simulink model "propellantmassfunction"  (R2025b)
settings: Solver=VariableStepAuto  StartTime=0.0  StopTime=10.0  RelTol=1e-3
settings Model: Creator=zachm  LastModifiedBy=zachm

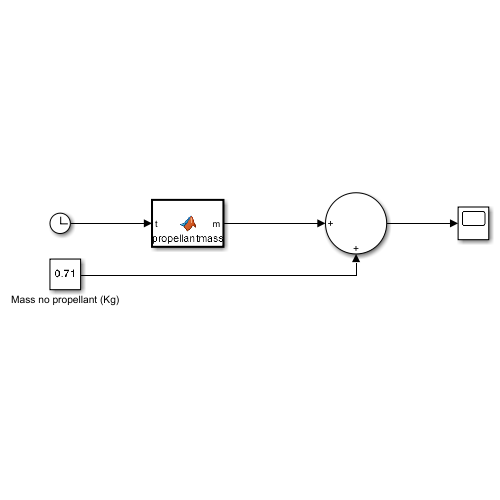
[thumbnail: Simulink's stored preview of the top-level diagram]
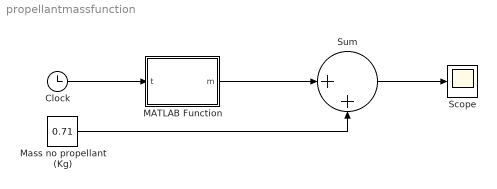
== system propellantmassfunction ==
  Clock : Clock
  MATLAB Function : MATLAB Function  TreatAsAtomicUnit=on
  Mass no propellant (Kg) : Constant  Value=0.71
  Scope : Scope
      settings: ActiveDisplayYMinimum=0.70985137869025383  ActiveDisplayYMaximum=0.72330515236022874
  Sum : Sum  Inputs=|++
  wires:
  Clock/1 -> MATLAB Function/1(t)
  MATLAB Function/1(m) -> Sum/1
  Mass no propellant (Kg)/1 -> Sum/2
  Sum/1 -> Scope/1

== matlab function propellantmassfunction/MATLAB Function ==
  data: t input; m output
function m = propellantmass(t)
    %#codegen
    m = ((0.3567 * t^2) - (8.072 *t) + 39.18)/1000;
    end
